simulink model "solverDiscStatesMultirate"  (R2018a)
settings: Solver=VariableStepDiscrete  StartTime=0.0  StopTime=20  RelTol=1e-3
settings Model: Creator=jrivitus  LastModifiedBy=bneiswan
settings DataIOCC: LimitDataPoints=on  SaveFormat=Array
settings OptimizationCC: ExpressionDepthLimit=2147483647  InitFltsAndDblsToZero=on  LifeSpan=inf
settings DebuggingCC: UnderspecifiedInitializationDetection=Classic  MergeDetectMultiDrivingBlocksExec=none  ParameterPrecisionLossMsg=none  FcnCallInpInsideContextMsg=warning  AllowSymbolicDim=off  StateNameClashWarn=warning  SFUnexpectedBacktrackingDiag=warning  SFNoUnconditionalDefaultTransitionDiag=warning  SFExecutionAtInitializationDiag=none
settings HardwareCC: ProdBitPerPointer=32  ProdBitPerSizeT=32  ProdBitPerPtrDiffT=32  ProdLargestAtomicFloat=None  ProdIntDivRoundTo=Undefined  ProdEndianess=Unspecified  ProdWordSize=32  ProdHWDeviceType=32-bit Generic
settings ModelReferenceCC: PropagateSignalLabelsOutOfModel=off
settings CodeAppCC: StateflowObjectComments=on
settings GRTTargetCC: TargetLangStandard=C89/C90 (ANSI)  GeneratePreprocessorConditionals=Disable all  CombineOutputUpdateFcns=off  GRTInterface=on
settings ConfigComp: CovMetricSettings=dw  CovHtmlReporting=on  CovSaveCumulativeToWorkspaceVar=on  CovSaveSingleToWorkspaceVar=on  CovExternalEMLEnable=off  CovSFcnEnable=off

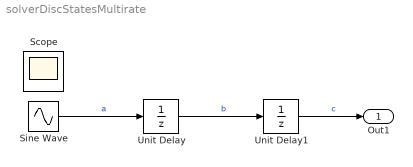
== system solverDiscStatesMultirate ==
  Sine Wave : Sin  SampleTime=0
  Unit Delay : UnitDelay  SampleTime=0.6
      settings: AttributesFormatString=|
      | Ts = %<SampleTime>
      | I.C. = %<InitialCondition>
  Unit Delay1 : UnitDelay  SampleTime=0.4
      settings: AttributesFormatString=|
      | Ts = %<SampleTime>
      | I.C. = %<InitialCondition>
  Out1 : Outport
  Scope : Scope
  wires:
  Sine Wave/1 -> Unit Delay/1  "a"
  Unit Delay1/1 -> Out1/1  "c"
  Unit Delay/1 -> Unit Delay1/1  "b"
